simulink model "rlc_notch_filter_differential_eq"  (R2020a)
settings: Solver=FixedStepAuto  StartTime=0.0  StopTime=duration  FixedStep=deltaT  RelTol=1e-3
values from neighbouring files (symbols this model uses):
  A = 1    [dataAnalisys.m]
  C = 1000*1e-6    (= 0.001)    [dataAnalisys.m]
  L = 1000*1e-3    (= 1)    [dataAnalisys.m]
  R = 1    [dataAnalisys.m]
  w = omega(i)    [dataAnalisys.m]
settings Model: Creator=acer  LastModifiedBy=acer

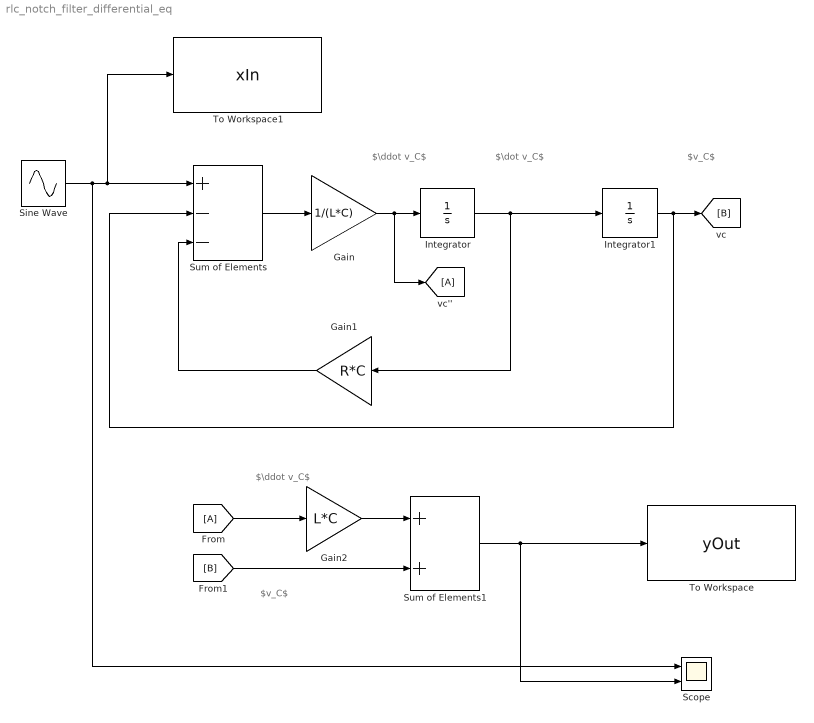
== system rlc_notch_filter_differential_eq ==
  note: $\ddot v_C$
  note: $\dot v_C$
  note: $v_C$
  note: $\ddot v_C$
  note: $v_C$
  Gain : Gain  Gain=1/(L*C)
  Gain1 : Gain  Gain=R*C
  Gain2 : Gain  Gain=L*C
  Integrator : Integrator
  Integrator1 : Integrator
  Scope : Scope  NumInputPorts=2
  Sine Wave : Sin  Amplitude=A  Frequency=w  SampleTime=0
  Sum of Elements : Sum  Inputs=+--
  Sum of Elements1 : Sum
  To Workspace : ToWorkspace  VariableName=yOut  SampleTime=-1
      settings: Save2DSignal=2-D array (concatenate along first dimension)
  To Workspace1 : ToWorkspace  VariableName=xIn  SampleTime=-1
      settings: Save2DSignal=2-D array (concatenate along first dimension)
  wires:
  Sum of Elements/1 -> Gain/1
  Gain/1 -> [A], Integrator/1
  Integrator/1 -> Gain1/1, Integrator1/1
  Sine Wave/1 -> Scope/1, To Workspace1/1, Sum of Elements/1
  Gain1/1 -> Sum of Elements/3
  Integrator1/1 -> Sum of Elements/2, [B]
  [A] -> Gain2/1
  Gain2/1 -> Sum of Elements1/1
  [B] -> Sum of Elements1/2
  Sum of Elements1/1 -> Scope/2, To Workspace/1
